simulink model "Simple_Controller"  (R2022a)
settings: Solver=ode15s  StartTime=0.0  StopTime=1  RelTol=1e-6  AbsTol=1e-6
values from neighbouring files (symbols this model uses):
  AN =     [MassIdentity_Test_SS_EIS_SOC50.mat]    (also in MassIdentity_Test_SS_EIS_SOC80.46.mat; Semi_Explicit_Test_KPCont_Profile_CV_Test_1SmallStepSOC81.93.mat; Semi_Explicit_Test_SS_EIS_SOC81.93.mat)
  CA =     [MassIdentity_Test_SS_EIS_SOC50.mat]    (also in MassIdentity_Test_SS_EIS_SOC80.46.mat; Semi_Explicit_Test_KPCont_Profile_CV_Test_1SmallStepSOC81.93.mat; Semi_Explicit_Test_SS_EIS_SOC81.93.mat)
  CONS =     [MassIdentity_Test_SS_EIS_SOC50.mat]    (also in MassIdentity_Test_SS_EIS_SOC80.46.mat; Semi_Explicit_Test_KPCont_Profile_CV_Test_1SmallStepSOC81.93.mat; Semi_Explicit_Test_SS_EIS_SOC81.93.mat)
  den = cell2mat(den)    [FullBatteryControl.m]    (also in FullBatteryControl_SS_Model.m)
  EL =     [MassIdentity_Test_SS_EIS_SOC50.mat]    (also in MassIdentity_Test_SS_EIS_SOC80.46.mat; Semi_Explicit_Test_KPCont_Profile_CV_Test_1SmallStepSOC81.93.mat; Semi_Explicit_Test_SS_EIS_SOC81.93.mat)
  FLAG =     [MassIdentity_Test_SS_EIS_SOC50.mat]    (also in MassIdentity_Test_SS_EIS_SOC80.46.mat; Semi_Explicit_Test_KPCont_Profile_CV_Test_1SmallStepSOC81.93.mat; Semi_Explicit_Test_SS_EIS_SOC81.93.mat)
  i_user_IC = 0    [FullBatteryControl.m]
  mass_inv = SIM.M_DiffEq_Inv    [FullBatteryControl.m]
  N =     [MassIdentity_Test_SS_EIS_SOC50.mat]    (also in MassIdentity_Test_SS_EIS_SOC80.46.mat; Semi_Explicit_Test_KPCont_Profile_CV_Test_1SmallStepSOC81.93.mat; Semi_Explicit_Test_SS_EIS_SOC81.93.mat)
  num = cell2mat(num)    [FullBatteryControl.m]    (also in FullBatteryControl_SS_Model.m)
  OutputMatrix = zeros(1,length(SIM.SV_IC))    [FullBatteryControl.m]
  P =     [MassIdentity_Test_SS_EIS_SOC50.mat]    (also in MassIdentity_Test_SS_EIS_SOC80.46.mat; Semi_Explicit_Test_KPCont_Profile_CV_Test_1SmallStepSOC81.93.mat; Semi_Explicit_Test_SS_EIS_SOC81.93.mat)
  PROPS = [100 0.28 0.00733702042142 0.6 2266 720 7.5e-11 1 0.363 3e-13 3e-13 3e-13 ... (475 elements, 19x25)]    [MassIdentity_Test_SS_EIS_SOC50.mat]    (also in MassIdentity_Test_SS_EIS_SOC80.46.mat; Semi_Explicit_Test_KPCont_Profile_CV_Test_1SmallStepSOC81.93.mat; Semi_Explicit_Test_SS_EIS_SOC81.93.mat)
  SEP =     [MassIdentity_Test_SS_EIS_SOC50.mat]    (also in MassIdentity_Test_SS_EIS_SOC80.46.mat; Semi_Explicit_Test_KPCont_Profile_CV_Test_1SmallStepSOC81.93.mat; Semi_Explicit_Test_SS_EIS_SOC81.93.mat)
  SIM = rmfield(SIM,'ControllerHandle')    [FullBatteryControl.m]    (also in FullBatteryControl_SS_Model.m = rmfield(SIM,'fsolve_options'); MassIdentity_Test_SS_EIS_SOC50.mat = ; MassIdentity_Test_SS_EIS_SOC80.46.mat = ; Semi_Explicit_Test_KPCont_Profile_CV_Test_1SmallStepSOC81.93.mat = )
  u_IC = SV_IC(SIM.Diff_idx)    [FullBatteryControl.m]
  v_IC = SV_IC(SIM.Algb_idx)    [FullBatteryControl.m]
settings Model: Creator=tyevans  LastModifiedBy=tyevans
settings DebuggingCC: AlgebraicLoopMsg=none  UnconnectedInputMsg=warning  UnconnectedOutputMsg=warning  UnconnectedLineMsg=warning  SFMachineParentedDataDiag=warning
settings RTWCC: DLArmComputeVersion=19.05

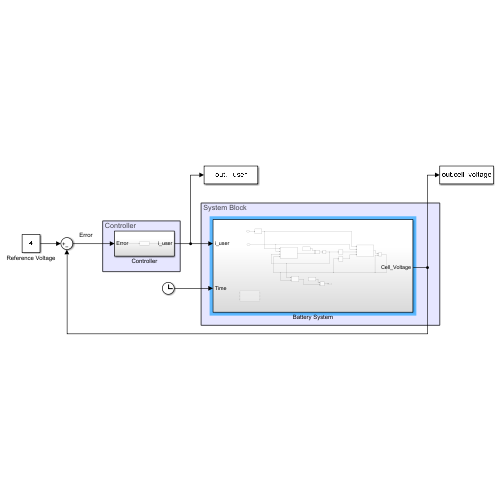
[thumbnail: Simulink's stored preview of the top-level diagram]
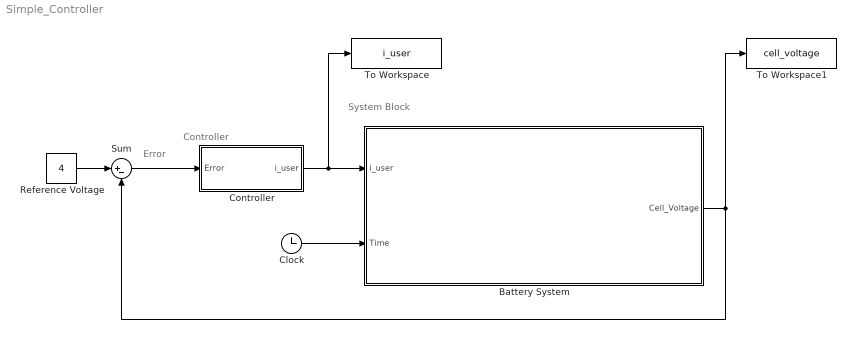
== system Simple_Controller ==
  note: Error
  note: System Block
  note: Controller
  Battery System : Subsystem
  Clock : Clock
  Controller : Subsystem
  Reference Voltage : Constant  Value=4
  Sum : Sum  Inputs=|+-
  To Workspace : ToWorkspace  VariableName=i_user  SampleTime=-1
  To Workspace1 : ToWorkspace  VariableName=cell_voltage  SampleTime=-1
  wires:
  Reference Voltage/1 -> Sum/1
  Battery System/1(Cell_Voltage) -> To Workspace1/1, Sum/2
  Controller/1(i_user) -> To Workspace/1, Battery System/1(i_user)
  Sum/1 -> Controller/1(Error)
  Clock/1 -> Battery System/2(Time)

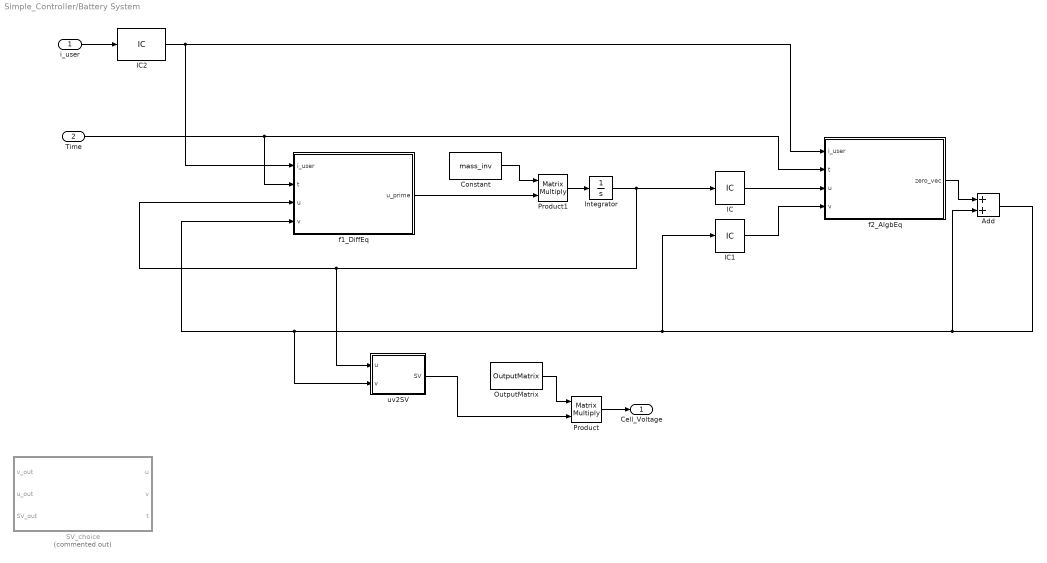
== system Simple_Controller/Battery System ==
  i_user : Inport
  Time : Inport  Port=2
  Add : Sum
  Constant : Constant  Value=mass_inv  VectorParams1D=off
  IC : InitialCondition  Value=u_IC
  IC1 : InitialCondition  Value=v_IC
  IC2 : InitialCondition  Value=i_user_IC
  Integrator : Integrator
  OutputMatrix : Constant  Value=OutputMatrix  VectorParams1D=off
  Product : Product  Multiplication=Matrix(*)
  Product1 : Product  Multiplication=Matrix(*)
  SV_choice : MATLAB Function  Commented=on  TreatAsAtomicUnit=on
  f1_DiffEq : MATLAB Function  TreatAsAtomicUnit=on
  f2_AlgbEq : MATLAB Function  TreatAsAtomicUnit=on
  uv2SV : MATLAB Function  TreatAsAtomicUnit=on
  Cell_Voltage : Outport
  wires:
  Time/1 -> f2_AlgbEq/2(t), f1_DiffEq/2(t)
  Product/1 -> Cell_Voltage/1
  OutputMatrix/1 -> Product/1
  Product1/1 -> Integrator/1
  Constant/1 -> Product1/1
  f1_DiffEq/1(u_prime) -> Product1/2
  f2_AlgbEq/1(zero_vec) -> Add/1
  i_user/1 -> IC2/1
  uv2SV/1(SV) -> Product/2
  IC2/1 -> f1_DiffEq/1(i_user), f2_AlgbEq/1(i_user)
  Integrator/1 -> IC/1, f1_DiffEq/3(u), uv2SV/1(u)
  Add/1 -> Add/2, IC1/1, f1_DiffEq/4(v), uv2SV/2(v)
  IC/1 -> f2_AlgbEq/3(u)
  IC1/1 -> f2_AlgbEq/4(v)

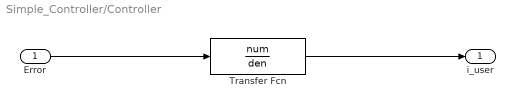
== system Simple_Controller/Controller ==
  Error : Inport
  Transfer Fcn : TransferFcn  Numerator=num  Denominator=den
  i_user : Outport
  wires:
  Transfer Fcn/1 -> i_user/1
  Error/1 -> Transfer Fcn/1

== matlab function Simple_Controller/Battery System/SV_choice ==
  data: v_out output size=[N.N_Algb , 1]; u input; v input; t input; u_out output size=[N.N_Diff , 1]; SIM parameter; N parameter; SV_out output size=[N.N_SV_tot,1]
function [v_out , u_out, SV_out] = SV_choice(u, v, t, SIM, N)
% Initialize Outputs
u_out  = zeros(length(SIM.Diff_idx),1);
v_out  = zeros(length(SIM.Algb_idx),1);
SV_out = zeros(N.N_SV_tot,1);

% If t = 0, then set u and v to IC
    if t == 0
        u_out  = SIM.SV_IC(SIM.Diff_idx);
        v_out  = SIM.SV_IC(SIM.Algb_idx);
        SV_out = SIM.SV_IC;
    else
        u_out = u;
        v_out = v;
        for i = 1:length(u)
            SV_out(SIM.Diff_idx(i)) = u(i);
        end
        for i = 1:length(v)
            SV_out(SIM.Algb_idx(i)) = v(i);
        end
    end
end

== matlab function Simple_Controller/Battery System/f1_DiffEq ==
  data: i_user input; t input; u input; v input; u_prime output size=[N.N_Diff , 1]; AN parameter; CA parameter; SEP parameter; EL parameter; SIM parameter; CONS parameter; P parameter; N parameter; FLAG parameter; PROPS parameter
function u_prime = f1_DiffEq(i_user, t, u, v, AN, CA, SEP, EL, SIM, CONS, P, N, FLAG, PROPS)
% Initialize output
u_prime = zeros(length(SIM.Diff_idx),1);

% Convert u and v to SV
% if t == 0
%     SV = SIM.SV_IC;
% else
    SV = zeros(N.N_SV_tot,1);
    for i = 1:length(u)
        SV(SIM.Diff_idx(i)) = u(i);
    end
    for i = 1:length(v)
        SV(SIM.Algb_idx(i)) = v(i);
    end
% end

% Call GovnEqns
coder.extrinsic('ConvertStrCallGov')
dSVdt = ConvertStrCallGov(t,SV,AN,CA,SEP,EL,SIM,CONS,P,N,FLAG,PROPS,i_user);

% Return just the differential variables
u_prime = dSVdt(SIM.Diff_idx);

end

== matlab function Simple_Controller/Battery System/f2_AlgbEq ==
  data: i_user input; t input; u input; v input; zero_vec output size=[N.N_Algb , 1]; AN parameter; CA parameter; SEP parameter; EL parameter; SIM parameter; CONS parameter; P parameter; N parameter; FLAG parameter; PROPS parameter
function zero_vec = f2_AlgbEq(i_user, t, u, v, AN, CA, SEP, EL, SIM, CONS, P, N, FLAG, PROPS)
% Initialize output
zero_vec = zeros(length(SIM.Algb_idx),1);

% Convert u and v to SV
% if t == 0
%     SV = SIM.SV_IC;
% else
    SV = zeros(N.N_SV_tot,1);
    for i = 1:length(u)
        SV(SIM.Diff_idx(i)) = u(i);
    end
    for i = 1:length(v)
        SV(SIM.Algb_idx(i)) = v(i);
    end
% end

 % Call GovnEqns
coder.extrinsic('ConvertStrCallGov')
dSVdt = ConvertStrCallGov(t,SV,AN,CA,SEP,EL,SIM,CONS,P,N,FLAG,PROPS,i_user);

% Return just the differential variables
zero_vec = dSVdt(SIM.Algb_idx);
t;
sum_zero_vec = sum(zero_vec);

end

== matlab function Simple_Controller/Battery System/uv2SV ==
  data: u input; SV output size=[N.N_SV_tot,1]; v input; SIM parameter; N parameter
function SV  = uv2SV(u,v, SIM, N)
SV = zeros(N.N_SV_tot,1);

for i = 1:length(u)
    SV(SIM.Diff_idx(i)) = u(i);
end
for i = 1:length(v)
    SV(SIM.Algb_idx(i)) = v(i);
end


end
